simulink library "Atmospheric_final"  (R2022b)
settings: Solver=VariableStepAuto  StartTime=0.0  StopTime=10.0  RelTol=1e-3
settings Model: Creator=Dell  LastModifiedBy=Dell

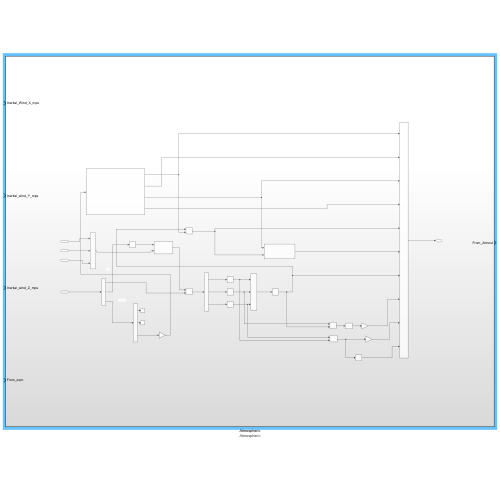
[thumbnail: Simulink's stored preview of the top-level diagram]
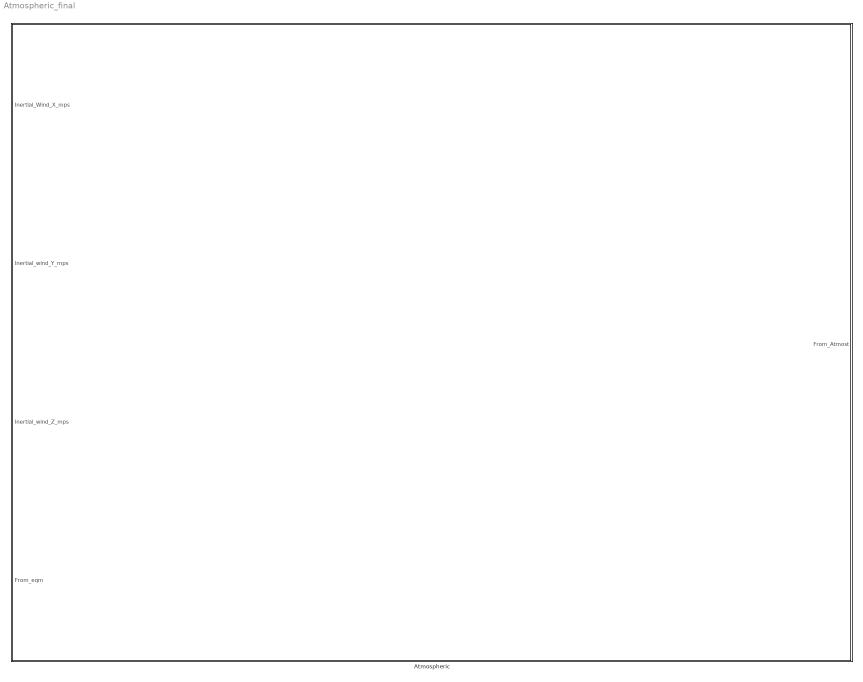
== system Atmospheric_final ==
  Atmospheric : Subsystem  Description=Atmospheric
      settings: AttributesFormatString=Atmospheric

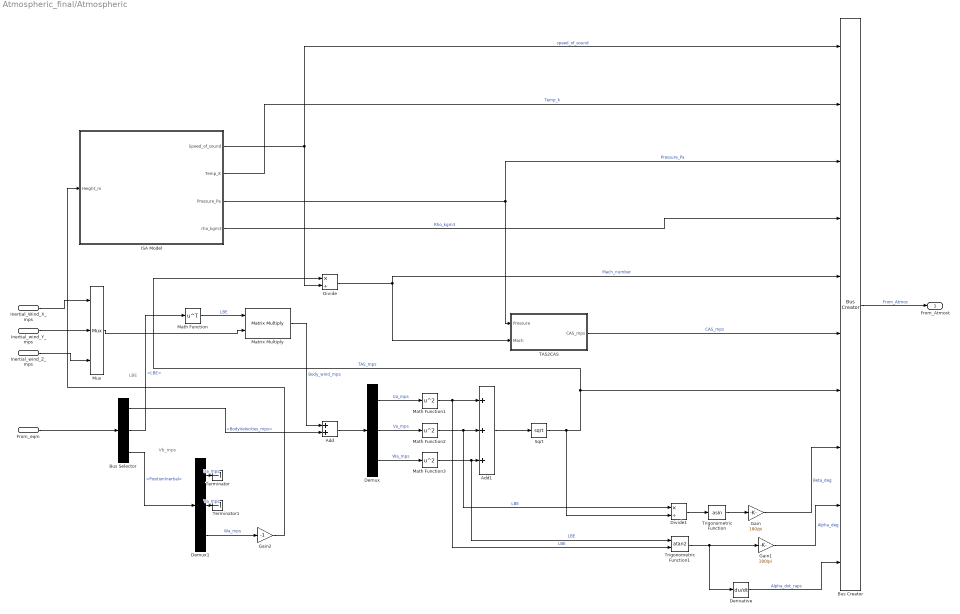
== system Atmospheric_final/Atmospheric ==
  note: Vb_mps
  note: LBE
  Inertial_Wind_X_mps : Inport
  Inertial_wind_Y_mps : Inport  Port=2
  Inertial_wind_Z_mps : Inport  Port=3
  From_eqm : Inport  Port=4
  Add : Sum
  Add1 : Sum  Inputs=+++
  Bus Creator : BusCreator  Inputs=10
  Bus Selector : BusSelector  OutputSignals=BodyVelocities_mps,LBE,PositionInertial
  Demux : Demux  Outputs=3
  Demux1 : Demux  Outputs=3
  Derivative : Derivative
  Divide : Product  Inputs=*/
  Divide1 : Product  Inputs=*/
  Gain : Gain  Gain=180/pi
  Gain1 : Gain  Gain=180/pi
  Gain2 : Gain  Gain=-1
  ISA Model : Subsystem
  Math Function : Math  Operator=transpose
  Math Function1 : Math  Operator=square
  Math Function2 : Math  Operator=square
  Math Function3 : Math  Operator=square
  Matrix Multiply : Product  Multiplication=Matrix(*)
  Mux : Mux  Inputs=3
  Sqrt : Sqrt
  TAS2CAS : Subsystem
  Terminator : Terminator
  Terminator1 : Terminator
  Trigonometric Function : Trigonometry  Operator=asin
  Trigonometric Function1 : Trigonometry  Operator=atan2
  From_Atmost : Outport
  wires:
  Demux1/3 -> Gain2/1  "Wa_mps"
  Demux1/2 -> Terminator1/1  "Va_mps"
  Demux1/1 -> Terminator/1  "Ua_mps"
  Bus Selector/3 -> Demux1/1  "<PositionInertial>"
  Bus Selector/1 -> Add/2  "<BodyVelocities_mps>"
  Bus Selector/2 -> Math Function/1  "<LBE>"
  Divide/1 -> TAS2CAS/2(Mach), Bus Creator/5  "Mach_number"
  Derivative/1 -> Bus Creator/10  "Alpha_dot_raps"
  Trigonometric Function/1 -> Gain/1
  Inertial_Wind_X_mps/1 -> Mux/1
  ISA Model/1(Speed_of_sound) -> Bus Creator/1, Divide/2  "speed_of_sound"
  Gain2/1 -> ISA Model/1(Height_m)
  Demux/2 -> Math Function2/1  "Va_mps"
  Trigonometric Function1/1 -> Derivative/1, Gain1/1
  Demux/3 -> Math Function3/1  "Wa_mps"
  Math Function2/1 -> Divide1/1, Add1/2  "LBE"
  Add/1 -> Demux/1
  ISA Model/3(Pressure_Pa) -> Bus Creator/3, TAS2CAS/1(Pressure)  "Pressure_Pa"
  Math Function/1 -> Matrix Multiply/1  "LBE"
  ISA Model/4(rho_kgm3) -> Bus Creator/4  "Rho_kgm3"
  Gain1/1 -> Bus Creator/9  "Alpha_deg"
  Math Function3/1 -> Trigonometric Function1/1, Add1/3  "LBE"
  ISA Model/2(Temp_K) -> Bus Creator/2  "Temp_k"
  Sqrt/1 -> Divide1/2, Bus Creator/7, Divide/1  "TAS_mps"
  Math Function1/1 -> Add1/1, Trigonometric Function1/2  "LBE"
  Inertial_wind_Z_mps/1 -> Mux/3
  Bus Creator/1 -> From_Atmost/1  "From_Atmos"
  Gain/1 -> Bus Creator/8  "Beta_deg"
  Inertial_wind_Y_mps/1 -> Mux/2
  Add1/1 -> Sqrt/1
  TAS2CAS/1(CAS_mps) -> Bus Creator/6  "CAS_mps"
  Divide1/1 -> Trigonometric Function/1
  Demux/1 -> Math Function1/1  "Ua_mps"
  Mux/1 -> Matrix Multiply/2
  From_eqm/1 -> Bus Selector/1
  Matrix Multiply/1 -> Add/1  "Body_wind_mps"

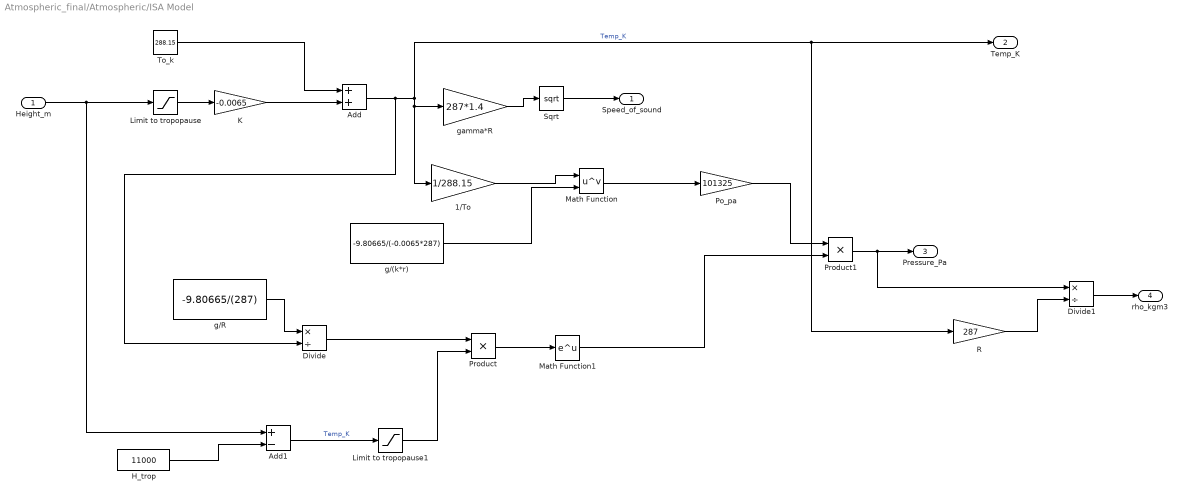
== system Atmospheric_final/Atmospheric/ISA Model ==
  Height_m : Inport
  1/To : Gain  Gain=1/288.15
  Add : Sum
  Add1 : Sum  Inputs=+-
  Divide : Product  Inputs=*/
  Divide1 : Product  Inputs=*/
  H_trop : Constant  Value=11000
  K : Gain  Gain=-0.0065
  Limit to tropopause : Saturate  UpperLimit=11000  LowerLimit=0
  Limit to tropopause1 : Saturate  UpperLimit=inf  LowerLimit=0
  Math Function : Math  Operator=pow
  Math Function1 : Math
  Po_pa : Gain  Gain=101325
  Product : Product
  Product1 : Product
  R : Gain  Gain=287
  Sqrt : Sqrt
  To_k : Constant  Value=288.15
  g/(k*r) : Constant  Value=-9.80665/(-0.0065*287)
  g/R : Constant  Value=-9.80665/(287)
  gamma*R : Gain  Gain=287*1.4
  Speed_of_sound : Outport
  Temp_K : Outport  Port=2
  Pressure_Pa : Outport  Port=3
  rho_kgm3 : Outport  Port=4
  wires:
  Math Function1/1 -> Product1/2
  R/1 -> Divide1/2
  g/R/1 -> Divide/1
  Product/1 -> Math Function1/1
  Product1/1 -> Pressure_Pa/1, Divide1/1
  K/1 -> Add/2
  Add/1 -> Divide/2, Temp_K/1, R/1, 1/To/1, gamma*R/1  "Temp_K"
  Math Function/1 -> Po_pa/1
  To_k/1 -> Add/1
  gamma*R/1 -> Sqrt/1
  1/To/1 -> Math Function/1
  g/(k*r)/1 -> Math Function/2
  Divide1/1 -> rho_kgm3/1
  Height_m/1 -> Add1/1, Limit to tropopause/1
  Po_pa/1 -> Product1/1
  Add1/1 -> Limit to tropopause1/1  "Temp_K"
  Limit to tropopause/1 -> K/1
  Sqrt/1 -> Speed_of_sound/1
  Limit to tropopause1/1 -> Product/2
  H_trop/1 -> Add1/2
  Divide/1 -> Product/1

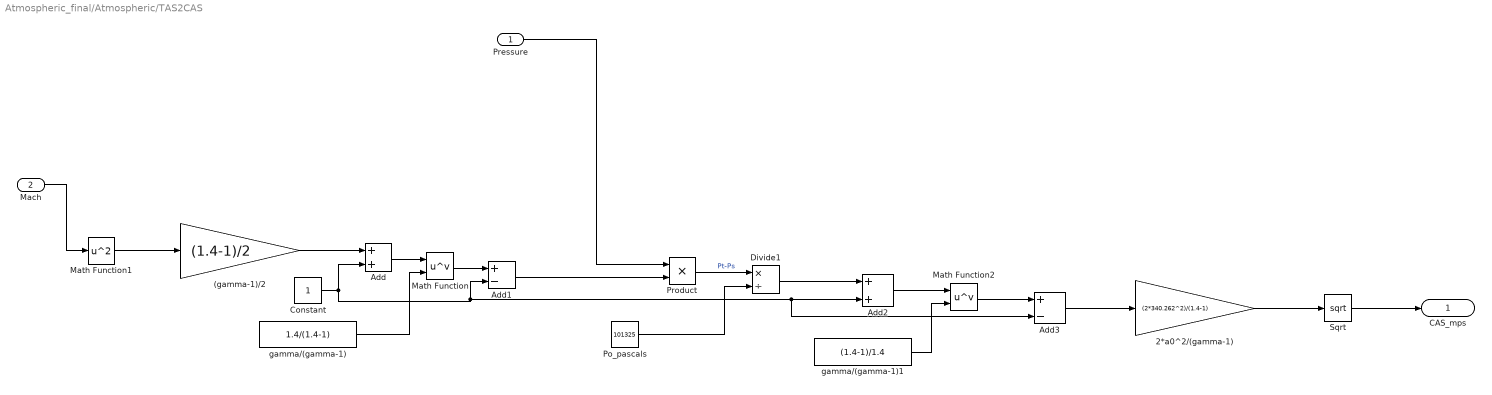
== system Atmospheric_final/Atmospheric/TAS2CAS ==
  Pressure : Inport
  Mach : Inport  Port=2
  (gamma-1)/2 : Gain  Gain=(1.4-1)/2
  2*a0^2/(gamma-1) : Gain  Gain=(2*340.262^2)/(1.4-1)
  Add : Sum
  Add1 : Sum  Inputs=+-
  Add2 : Sum
  Add3 : Sum  Inputs=+-
  Constant : Constant
  Divide1 : Product  Inputs=*/
  Math Function : Math  Operator=pow
  Math Function1 : Math  Operator=square
  Math Function2 : Math  Operator=pow
  Po_pascals : Constant  Value=101325
  Product : Product
  Sqrt : Sqrt
  gamma/(gamma-1) : Constant  Value=1.4/(1.4-1)
  gamma/(gamma-1)1 : Constant  Value=(1.4-1)/1.4
  CAS_mps : Outport
  wires:
  Po_pascals/1 -> Divide1/2
  Constant/1 -> Add/2, Add3/2, Add2/2, Add1/2
  Sqrt/1 -> CAS_mps/1
  Add3/1 -> 2*a0^2/(gamma-1)/1
  gamma/(gamma-1)1/1 -> Math Function2/2
  Pressure/1 -> Product/1
  (gamma-1)/2/1 -> Add/1
  Math Function/1 -> Add1/1
  gamma/(gamma-1)/1 -> Math Function/2
  Divide1/1 -> Add2/1
  Product/1 -> Divide1/1  "Pt-Ps"
  Add/1 -> Math Function/1
  Math Function1/1 -> (gamma-1)/2/1
  2*a0^2/(gamma-1)/1 -> Sqrt/1
  Math Function2/1 -> Add3/1
  Add1/1 -> Product/2
  Add2/1 -> Math Function2/1
  Mach/1 -> Math Function1/1
